simulink model "fullfilterxyz"  (R2019b)
settings: Solver=ode3  StartTime=0.0  StopTime=100  FixedStep=1  RelTol=1e-3
libraries: aerolibconvert2 x3, sharedutil x3, sharedtransform x3, simulink x1
settings Model: Creator=pieterpinson  LastModifiedBy=pieterpinson
settings DataIOCC: SaveFormat=StructureWithTime
settings OptimizationCC: LifeSpan=inf
settings DebuggingCC: SFExecutionAtInitializationDiag=none  ArithmeticOperatorsInVariantConditions=warning
settings HardwareCC: ProdBitPerSizeT=32  ProdBitPerPtrDiffT=32  ProdWordSize=32  ProdHWDeviceType=Specified
settings SFSimCC: CustomCodeUndefinedFunction=UseInterfaceOnly
settings CodeAppCC: StateflowObjectComments=on

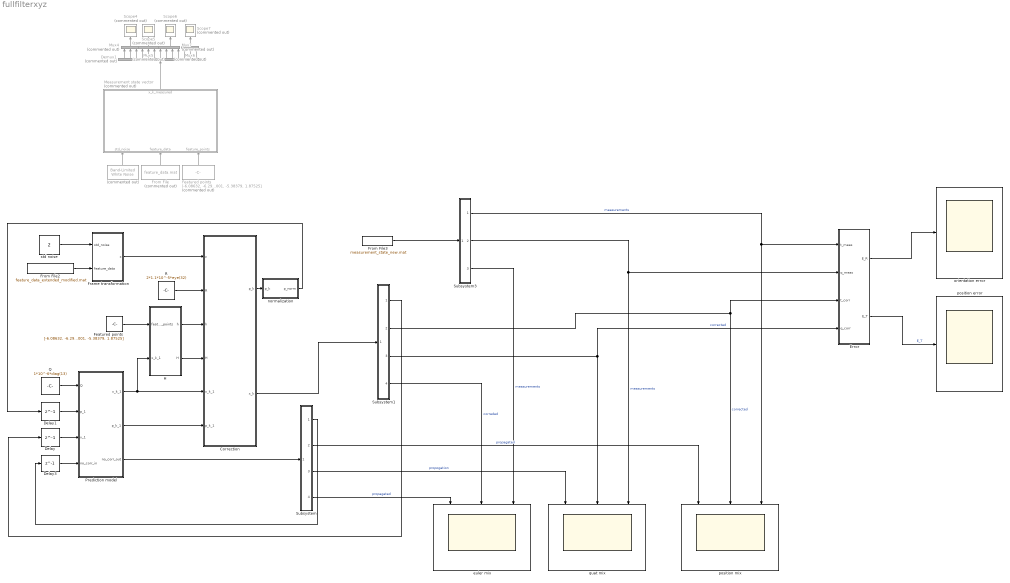
== system fullfilterxyz ==
  "       " : simulink/Sources/Band-Limited White Noise  Commented=on  Cov=0  Ts=1  seed=[23341]
  " position error" : Scope
  Correction : MATLAB Function  TreatAsAtomicUnit=on
  Delay : Delay  DelayLength=1  InitialCondition=[1 ;1; 148 ;0 ; 0 ; 0 ; -0.1013 ;-0.7516; -0.6013 ;-0.2516; -0.0873 ; -0.1489 ; 0.0262]
  Delay1 : Delay  DelayLength=1  InitialCondition=0.1*diag([1,1,1,1*10^-2,1*10^-2,1*10^-2,1*10^-5,1*10^-5,1*10^-5,1*10^-5,0.1,0.1,0.1])
  Delay3 : Delay  DelayLength=1  InitialCondition=[0 ; 0; 150; 0 ; 0 ; 0 ;0.1664; 0.7399; 0.6209; 0.1983; -0.0873 ; -0.1489 ; 0.0262]
  Demux1 : Demux  Commented=on  Outputs=13
  Error : MATLAB Function  TreatAsAtomicUnit=on
  Featured points : Constant  Value=|
      | [-6.08632, -6.29117, -6.23068, -6.170180, 0.66541, 0.66541, 2.50061, 2.48017, 6.23068, 6.35166, 6.35166, 6.29117,10.84578, 10.82807, 29.52664, 29.55825 ;
      | -0.63573, 1.88967, -0.6022, 1.85389, 2.17147, 2.18343, 3.10581, 3.09464, -0.6368, 2.53604, -0.62563, 2.54752, 2.60307, 1.32946, -8.00742, -9.30518 ;
      | -1.81476, -1.81476, 1.87525, 1.93574, 7.31953, -7.38003, -7.25904, 7.31953, 1.93574, 2.05673, -1.81476, -1.93574, -3.56903, 3.69001, -5.38379, 1.87525]
  "Featured points     " : Constant  Commented=on  Value=|
      | [-6.08632, -6.29117, -6.23068, -6.170180, 0.66541, 0.66541, 2.50061, 2.48017, 6.23068, 6.35166, 6.35166, 6.29117,10.84578, 10.82807, 29.52664, 29.55825 ;
      | -0.63573, 1.88967, -0.6022, 1.85389, 2.17147, 2.18343, 3.10581, 3.09464, -0.6368, 2.53604, -0.62563, 2.54752, 2.60307, 1.32946, -8.00742, -9.30518 ;
      | -1.81476, -1.81476, 1.87525, 1.93574, 7.31953, -7.38003, -7.25904, 7.31953, 1.93574, 2.05673, -1.81476, -1.93574, -3.56903, 3.69001, -5.38379, 1.87525]
  Frame transformation : MATLAB Function  TreatAsAtomicUnit=on
  From File : FromFile  Commented=on  FileName=feature_data.mat  SampleTime=1
  From File2 : FromFile  FileName=feature_data_extended_modified.mat  SampleTime=1
  From File3 : FromFile  FileName=measurement_state_new.mat  SampleTime=1
  H : MATLAB Function  TreatAsAtomicUnit=on
  Measurement state vector : MATLAB Function  Commented=on  TreatAsAtomicUnit=on
  Mux4 : Mux  Commented=on  Inputs=3
  Mux5 : Mux  Commented=on  Inputs=3
  Mux6 : Mux  Commented=on  Inputs=3
  Mux7 : Mux  Commented=on
  Prediction model : MATLAB Function  TreatAsAtomicUnit=on
  Q : Constant  Value=1*10^-6*diag(13)
  R : Constant  Value=2*1.1*10^-5*eye(32)
  Scope{4..7} (4 alike) : Scope  Commented=on
  Subsystem : Subsystem
  Subsystem1 : Subsystem
  Subsystem3 : Subsystem
  "euler mix " : Scope  NumInputPorts=3
  normalization : MATLAB Function  TreatAsAtomicUnit=on
  orientation error : Scope
  position mix : Scope  NumInputPorts=3
  quat mix : Scope  NumInputPorts=3
  std noise : Constant  Value=2
  wires:
  Prediction model/1(x_k_1) -> Correction/5(x_k_1), H/2(x_k_1)
  Delay/1 -> Prediction model/3(x_1)
  Q/1 -> Prediction model/1(Q)
  Delay1/1 -> Prediction model/2(p_1)
  Mux6/1 -> Scope7/1
  Demux1/3 -> Mux4/3
  Demux1/10 -> Mux7/4
  Demux1/2 -> Mux4/2
  Demux1/1 -> Mux4/1
  Demux1/11 -> Mux6/1
  Mux4/1 -> Scope4/1
  Mux5/1 -> Scope5/1
  Mux7/1 -> Scope6/1
  Demux1/6 -> Mux5/3
  Demux1/9 -> Mux7/3
  Demux1/13 -> Mux6/3
  Demux1/12 -> Mux6/2
  Demux1/7 -> Mux7/1
  Frame transformation/1(z) -> Correction/1(z)
  Demux1/4 -> Mux5/1
  Demux1/5 -> Mux5/2
  Demux1/8 -> Mux7/2
  Prediction model/2(p_k_1) -> Correction/6(p_k_1)
  R/1 -> Correction/2(R)
  std noise/1 -> Frame transformation/1(std_noise)
  Featured points/1 -> H/1(feature_points)
  Delay3/1 -> Prediction model/4(no_corr_in)
  Prediction model/3(no_corr_out) -> Subsystem/1(In1)
  Subsystem/1(Out1) -> Delay3/1
  Subsystem/2(Out2) -> position mix/1  "propagated"
  Subsystem/3(Out4) -> quat mix/1  "propogation"
  Subsystem/4(Out6) -> "euler mix "/1  "propagated"
  Correction/2(x_k) -> Subsystem1/1(In1)
  Subsystem1/1(Out1) -> Delay/1
  Subsystem1/4(Out6) -> "euler mix "/2  "correded"
  Measurement state vector/1(x_k_measured) -> Demux1/1
  Subsystem3/1(Out2) -> position mix/3, Error/1(t_meas)  "measurements"
  Subsystem3/3(Out6) -> "euler mix "/3  "measurements"
  From File/1 -> Measurement state vector/2(feature_data)
  From File2/1 -> Frame transformation/2(feature_data)
  Error/2(E_T) -> " position error"/1  "E_T"
  H/2(H) -> Correction/4(H)
  "Featured points     "/1 -> Measurement state vector/3(feature_points)
  "       "/1 -> Measurement state vector/1(std_noise)
  Subsystem3/2(Out4) -> quat mix/3, Error/2(q_meas)  "measurements"
  Subsystem1/3(Out4) -> Error/4(q_corr), quat mix/2  "corrected"
  From File3/1 -> Subsystem3/1(In1)
  Subsystem1/2(Out2) -> Error/3(t_corr), position mix/2  "corrected"
  Error/1(E_R) -> orientation error/1
  Correction/1(p_k) -> normalization/1(p_k)
  H/1(h) -> Correction/3(h)
  normalization/1(p_norm) -> Delay1/1

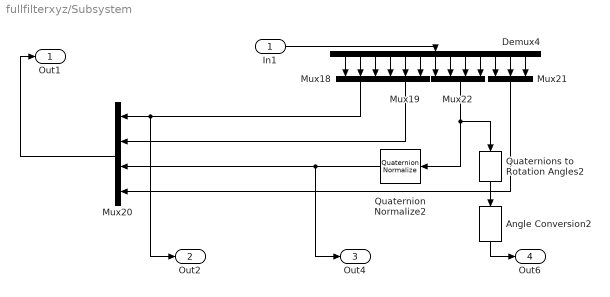
== system fullfilterxyz/Subsystem ==
  In1 : Inport
  Angle Conversion2 : aerolibconvert2/Angle Conversion  IU=rad  OU=deg
  Demux4 : Demux  Outputs=13
  Mux18 : Mux  Inputs=3
  Mux19 : Mux  Inputs=3
  Mux20 : Mux
  Mux21 : Mux  Inputs=3
  Mux22 : Mux
  Quaternion Normalize2 : sharedutil/Quaternion Normalize  aMode=aMode
      settings: SourceProductName=Aerospace Blockset  SourceProductBaseCode=AE
  Quaternions to Rotation Angles2 : sharedtransform/Quaternions to Rotation Angles  rotationOrder=ZYX  aMode=aMode
      settings: SourceProductBaseCode=AE
  Out1 : Outport
  Out2 : Outport  Port=2
  Out4 : Outport  Port=3
  Out6 : Outport  Port=4
  wires:
  Mux21/1 -> Mux20/4
  Mux22/1 -> Quaternion Normalize2/1, Quaternions to Rotation Angles2/1
  Demux4/13 -> Mux21/3
  Demux4/8 -> Mux22/2
  Demux4/1 -> Mux18/1
  Quaternion Normalize2/1 -> Out4/1, Mux20/3
  Mux19/1 -> Mux20/2
  Demux4/10 -> Mux22/4
  Demux4/5 -> Mux19/2
  Demux4/11 -> Mux21/1
  Demux4/2 -> Mux18/2
  Demux4/7 -> Mux22/1
  Demux4/12 -> Mux21/2
  Mux18/1 -> Out2/1, Mux20/1
  Demux4/3 -> Mux18/3
  Quaternions to Rotation Angles2/1 -> Angle Conversion2/1
  Demux4/9 -> Mux22/3
  Demux4/4 -> Mux19/1
  Demux4/6 -> Mux19/3
  In1/1 -> Demux4/1
  Mux20/1 -> Out1/1
  Angle Conversion2/1 -> Out6/1

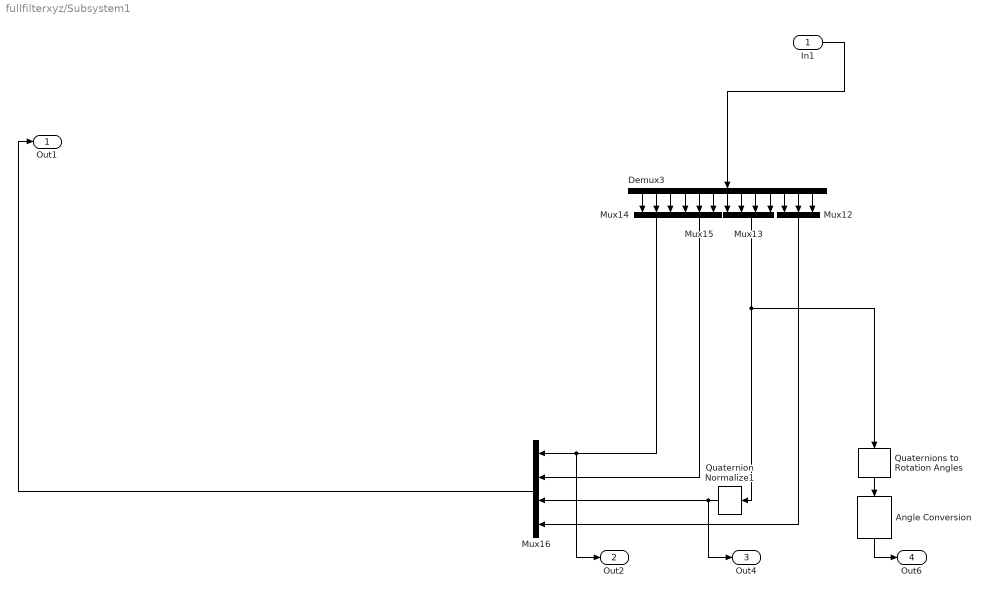
== system fullfilterxyz/Subsystem1 ==
  In1 : Inport
  Angle Conversion : aerolibconvert2/Angle Conversion  IU=rad  OU=deg
  Demux3 : Demux  Outputs=13
  Mux12 : Mux  Inputs=3
  Mux13 : Mux
  Mux14 : Mux  Inputs=3
  Mux15 : Mux  Inputs=3
  Mux16 : Mux
  Quaternion Normalize1 : sharedutil/Quaternion Normalize  aMode=aMode
      settings: SourceProductName=Aerospace Blockset  SourceProductBaseCode=AE
  Quaternions to Rotation Angles : sharedtransform/Quaternions to Rotation Angles  rotationOrder=ZYX  aMode=aMode
      settings: SourceProductBaseCode=AE
  Out1 : Outport
  Out2 : Outport  Port=2
  Out4 : Outport  Port=3
  Out6 : Outport  Port=4
  wires:
  Mux15/1 -> Mux16/2
  Demux3/2 -> Mux14/2
  Mux14/1 -> Out2/1, Mux16/1
  Quaternion Normalize1/1 -> Out4/1, Mux16/3
  Quaternions to Rotation Angles/1 -> Angle Conversion/1
  In1/1 -> Demux3/1
  Mux13/1 -> Quaternions to Rotation Angles/1, Quaternion Normalize1/1
  Demux3/8 -> Mux13/2
  Demux3/1 -> Mux14/1
  Demux3/4 -> Mux15/1
  Mux12/1 -> Mux16/4
  Demux3/7 -> Mux13/1
  Demux3/6 -> Mux15/3
  Demux3/3 -> Mux14/3
  Demux3/5 -> Mux15/2
  Demux3/11 -> Mux12/1
  Demux3/9 -> Mux13/3
  Demux3/10 -> Mux13/4
  Demux3/12 -> Mux12/2
  Demux3/13 -> Mux12/3
  Mux16/1 -> Out1/1
  Angle Conversion/1 -> Out6/1

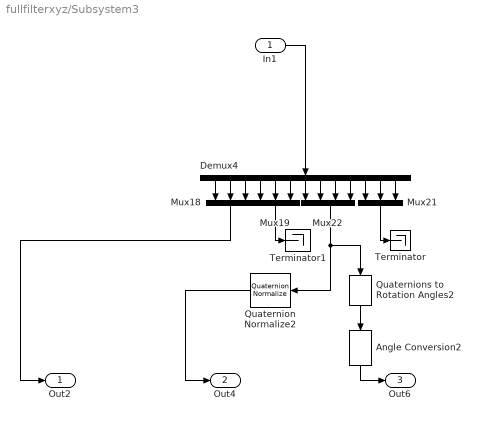
== system fullfilterxyz/Subsystem3 ==
  In1 : Inport
  Angle Conversion2 : aerolibconvert2/Angle Conversion  IU=rad  OU=deg
  Demux4 : Demux  Outputs=13
  Mux18 : Mux  Inputs=3
  Mux19 : Mux  Inputs=3
  Mux21 : Mux  Inputs=3
  Mux22 : Mux
  Quaternion Normalize2 : sharedutil/Quaternion Normalize  aMode=aMode
      settings: SourceProductName=Aerospace Blockset  SourceProductBaseCode=AE
  Quaternions to Rotation Angles2 : sharedtransform/Quaternions to Rotation Angles  rotationOrder=ZYX  aMode=aMode
      settings: SourceProductBaseCode=AE
  Terminator : Terminator
  Terminator1 : Terminator
  Out2 : Outport
  Out4 : Outport  Port=2
  Out6 : Outport  Port=3
  wires:
  Mux22/1 -> Quaternion Normalize2/1, Quaternions to Rotation Angles2/1
  Demux4/13 -> Mux21/3
  Demux4/8 -> Mux22/2
  Demux4/1 -> Mux18/1
  Quaternion Normalize2/1 -> Out4/1
  Demux4/10 -> Mux22/4
  Demux4/5 -> Mux19/2
  Demux4/11 -> Mux21/1
  Demux4/2 -> Mux18/2
  Demux4/7 -> Mux22/1
  Demux4/12 -> Mux21/2
  Mux18/1 -> Out2/1
  Demux4/3 -> Mux18/3
  Quaternions to Rotation Angles2/1 -> Angle Conversion2/1
  Demux4/9 -> Mux22/3
  Demux4/4 -> Mux19/1
  Demux4/6 -> Mux19/3
  In1/1 -> Demux4/1
  Angle Conversion2/1 -> Out6/1
  Mux19/1 -> Terminator1/1
  Mux21/1 -> Terminator/1

== matlab function fullfilterxyz/Frame transformation ==
  data: z output; std_noise input; feature_data input
function z = measurements(std_noise,feature_data)
   
    %import and convert featured data points 
    datapoints = feature_data(:,1);
    z = zeros(32,1);
    
    pixel_size = 1.1*10^-5;
    
    %number of featurepoints
    n = 16;
    
    for i=1:2*n
        
        z(i,1) = pixel_size*(datapoints(i) + std_noise);

    end
    
end

== matlab function fullfilterxyz/Prediction model ==
  data: x_k_1 output; Q input; p_1 input; p_k_1 output; x_1 input; no_corr_in input; no_corr_out output
function [x_k_1,p_k_1,no_corr_out]= prediction(Q,p_1,x_1,no_corr_in)

%x_k_1 = x_1;

%orbital parameter
mu = 3.986*10^14;
R_earth = 6371000;
H_target = 773000;
a = R_earth + H_target;
n = sqrt(mu/(a^3));

%clohessy-wiltshire equations
dr = [4-3*cos(n) 0 0 sin(n)/n 2*(1-cos(n))/n 0 ; 6*(sin(n)-n) 1 0 2*(cos(n)-1)/n (4*sin(n)-3*n)/n 0 ; 0 0 cos(n) 0 0 sin(n)/n];
dv = [3*n*sin(n) 0 0 cos(n) 2*sin(n) 0 ; 6*n*(cos(n)-1) 0 0 -2*sin(n) 4*cos(n)-3 0 ; 0 0 -n*sin(n) 0 0 cos(n)];
%phi = [dr;dv];

%quaternion kinematic equation
%dq = 0.5*[0 x_1(13) -x_1(12) x_1(11) ; -x_1(13) 0 x_1(11) x_1(12) ; x_1(12) -x_1(11) 0 x_1(13) ; -x_1(11) -x_1(12) -x_1(13) 0];
wq = eul2quat(x_1(11:13)','XYZ'); % This is the unit quaternion rotation due to omega
wq1 = [0.9962 ; -0.0445 ; -0.0737 ; 0.0163];
dq = [wq(1) -wq(2) -wq(3) -wq(4) ; wq(2) wq(1) wq(4) -wq(3) ; wq(3) -wq(4) wq(1) wq(2) ; wq(4) wq(3) -wq(2) wq(1)];
dq1 = [wq1(1) -wq1(2) -wq1(3) -wq1(4) ; wq1(2) wq1(1) wq1(4) -wq1(3) ; wq1(3) -wq1(4) wq1(1) wq1(2) ; wq1(4) wq1(3) -wq1(2) wq1(1)];

%x_k_1(1:6) = phi*x_1(1:6);
%x_k_1(7:10) = quatnormalize(quatmultiply(x_1(7:10)',dq1))';
%state transition matrix
fi = [dr zeros(3,7) ; dv zeros(3,7) ; zeros(4,6) dq zeros(4,3) ; zeros(3,10) eye(3)];
phi = [dr zeros(3,7) ; dv zeros(3,7) ; zeros(4,6) dq1 zeros(4,3) ; zeros(3,10) eye(3)];


%propogation step
%x_k_1 = [0;0;0;0;0;0;x_1(7:10);0;0;0] + fi * x_1;
x_k_1 = fi * x_1;
p_k_1 = fi * p_1 * fi.' + Q;
no_corr_out = phi * no_corr_in;
end


%dq1 = 0.5*[x_1(10) -x_1(9) x_1(8) x_1(7) ; x_1(9) x_1(10) -x_1(7) x_1(8) ; -x_1(8) x_1(7) x_1(10) x_1(9) ; -x_1(7) -x_1(8) -x_1(9) x_1(10)];
%fi(7,7) = x_1(7) + 0.5*(x_1(12)*x_1(8) - x_1(12)*x_1(9) + x_1(11)*x_1(10));
%fi(8,8) = x_1(8) + 0.5*(-x_1(13)*x_1(7) + x_1(11)*x_1(9) + x_1(12)*x_1(10));
%fi(9,9) = x_1(9) + 0.5*(x_1(12)*x_1(7) - x_1(11)*x_1(8) + x_1(13)*x_1(10));
%fi(10,10) = x_1(10) + 0.5*(-x_1(11)*x_1(7) - x_1(12)*x_1(8) - x_1(13)*x_1(9));

== matlab function fullfilterxyz/Correction ==
  data: z input; R input; h input; p_k output; x_k output; H input; x_k_1 input; p_k_1 input
function [p_k,x_k]= correction(z,R,h,H,x_k_1,p_k_1)

%kalman gain calculation
K = p_k_1 * H' * inv(H * p_k_1 * H' + R);

%correction step
x_k = x_k_1 + K*(z - h);
p_k = (eye(13,13) - K*H)*p_k_1;

end

== matlab function fullfilterxyz/H ==
  data: feature_points input; h output; x_k_1 input; H output
function [h,H]= Jacobian(feature_points,x_k_1)
    
    %focal length of the camera
    fx = 2*3.9*10^-3;
    fy = 2*3.9*10^-3;
    
    pixel_size = 1.1*10^-5;
    
    %number of featurepoints
    n = 16;

    %individual vector definition
    vectorJacobian = zeros(2*n, 3);
    quaternionJacobian = zeros(2*n, 4);
    h = zeros(32,1);
    
    %import and convert featured data points
    wireframe = feature_points;
    
    for i = 1:n
        
        %quaternion rotation matrix
        q = x_k_1(7:10);
        %R_q = [q(1)^2+q(2)^2-q(3)^2-q(3)^2 2*(q(2)*q(3)-q(1)*q(4)) 2*(q(4)*q(2)+q(1)*q(3));
         %2*(q(2)*q(3)+q(1)*q(4)) q(1)^2-q(2)^2+q(3)^2-q(4)^2 2*(q(3)*q(4)-q(1)*q(2));
         %2*(q(4)*q(2)-q(1)*q(3)) 2*(q(3)*q(4)+q(1)*q(2)) q(1)^2-q(2)^2-q(3)^2+q(4)^2];
        R_q = quat2rotm(q');
         
        %position vector
        xyz = R_q* wireframe(:,i)+ x_k_1(1:3);
        
        %h vector calculation
        h(2*i-1,1) = xyz(1)/xyz(3)*fx + 256*pixel_size;
        h(2*i,1) = xyz(2)/xyz(3)*fy + 256*pixel_size;
        
        %position Jacobian calculation
        vectorJacobian(i*2-1:i*2,1:3) = [fx/xyz(3) 0 -fx*xyz(1)/xyz(3)^2 ; 0 fy/xyz(3) -fy*xyz(2)/xyz(3)^2];
        
        %quaternion rotation Jacobian calculation
        dH_dq_1 = [2*q(1) -2*q(4) 2*q(3); 2*q(4) 2*q(1) -2*q(2); -2*q(3) 2*q(2) 2*q(1)]*xyz;
        dH_dq_2 = [2*q(2) 2*q(3) 2*q(4); 2*q(3) -2*q(2) -2*q(1); 2*q(4) 2*q(1) -2*q(2)]*xyz;
        dH_dq_3 = [-2*q(3) 2*q(2) 2*q(1); 2*q(2) 2*q(3) 2*q(4); -2*q(1) 2*q(4) -2*q(3)]*xyz;
        dH_dq_4 = [-2*q(4) -2*q(1) 2*q(2); 2*q(1) -2*q(4) 2*q(3); 2*q(1) 2*q(3) 2*q(4)]*xyz;
        dH_dq = [dH_dq_1 dH_dq_2 dH_dq_3 dH_dq_4] * [1 0 0 0; 0 -1 0 0; 0 0 -1 0; 0 0 0 -1];
        
        quaternionJacobian(i*2-1:i*2,1:4) = vectorJacobian(i*2-1:i*2,1:3)*dH_dq;
        
    end
    
    %final Jacobian vector
    H = [vectorJacobian, zeros(2*n, 3), quaternionJacobian, zeros(2*n, 3)];

end

== matlab function fullfilterxyz/Error ==
  data: t_meas input; q_meas input; t_corr input; E_R output; q_corr input; E_T output
function [E_R,E_T] = error(t_meas,q_meas,t_corr,q_corr)

    Beta = quatmultiply(q_meas', q_corr');
     
    E_T = abs(t_meas - t_corr);
    E_R = 2*acos(abs(Beta(1)));

end

== matlab function fullfilterxyz/Measurement state vector ==
  data: std_noise input; x_k_measured output; feature_data input; feature_points input
function x_k_measured = measurementstate(std_noise,feature_data,feature_points)

addpath EPnP;

    %focal length of the camera
    fx = 2*3.9*10^-3;
    fy = 2*3.9*10^-3;
    
    %number of featurepoints
    n = 16;
    
    %import and convert featured data points 
    datapoints = feature_data(:,1) + std_noise;
    
    %pixel size & number
    m = 1.1*10^-5;

    A=[fx/m 0 u0; 0 fy/m v0; 0 0 1];
    x3d_h=zeros(n,4);
    x2d_h=zeros(n,3); 
    
for i=1:n
    x3d_h(i,1:3) = feature_points(:,i)';
    x3d_h(i,4) = 1;
    x2d_h(i,1) = datapoints(2*i-1);
    x2d_h(i,2) = datapoints(2*i);
    x2d_h(i,3) = 1;
end

x_k_measured = EPnP2state_vector(x3d_h,x2d_h,A);

end

== matlab function fullfilterxyz/normalization ==
  data: p_k input; p_norm output
function p_norm = norm(p_k)
    
    q = [p_k(7,7) ; p_k(8,8) ; p_k(9,9) ; p_k(10,10)];
    
    qrot = [q(2)^2+q(3)^2+q(4)^2 , -q(1)*q(2), -q(1)*q(3), -q(1)*q(4) ; -q(2)*q(1), q(1)^2+q(3)^2+q(4)^2, -q(2)*q(3), -q(2)*q(4) ; -q(3)*q(1), -q(3)*q(2), q(1)^2+q(2)^2+q(4)^2, -q(3)*q(4) ; -q(4)*q(1), -q(4)*q(2), -q(4)*q(3), q(1)^2+q(2)^2+q(3)^2];

    dqnorm = (q(1)^2 + q(2)^2 + q(3)^2 + q(4)^2)^(-3/2) * qrot;

    J = [eye(6) zeros(6,7) ; zeros(4,6) dqnorm zeros(4,3); zeros(3,10) eye(3)];
    
    p_norm = J * p_k * J';

end
